simulink model "kalmannonlinear_noiseadded"  (R2019b)
settings: Solver=VariableStepAuto  StartTime=0.0  StopTime=10.0  RelTol=1e-3
libraries: sharedTrackingLibrary x9
settings Model: Creator=Bekircan Keceoglu  LastModifiedBy=Bekircan Keceoglu

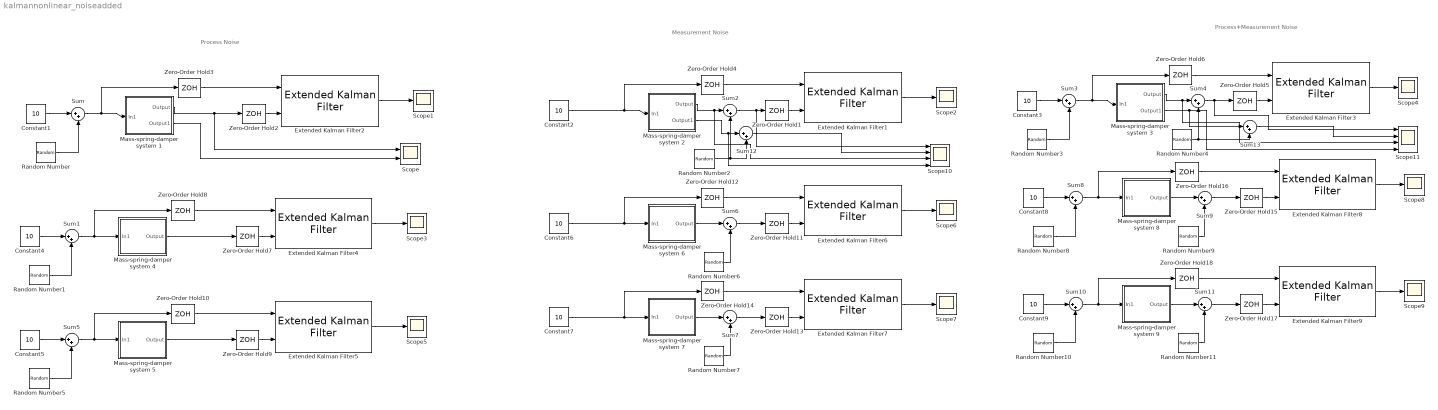
== system kalmannonlinear_noiseadded ==
  note: Process Noise
  note: Measurement Noise
  note: Process+Measurement Noise
  Constant{1..9} (9 alike) : Constant  Value=10
  Extended Kalman Filter1 : sharedTrackingLibrary/Extended Kalman Filter  StateTransitionFcn=myStateTransitionFcn  HasStateTransitionJacobianFcn=off  HasAdditiveProcessNoise=Additive  ProcessNoise=1  HasTimeVaryingProcessNoise=off  HasStateTransitionFcnExtraArgument=1  InitialState=[0 0]  InitialStateCovariance=1  MeasurementFcn1=myMeasurementFcn  HasMeasurementJacobianFcn1=off  HasMeasurementEnablePort1=off  HasAdditiveMeasurementNoise1=Additive  MeasurementNoise1=1  HasTimeVaryingMeasurementNoise1=off  HasMeasurementFcnExtraArgument1=0  MeasurementFcn2=myMeasurementFcn  HasMeasurementJacobianFcn2=off  HasMeasurementEnablePort2=off  HasAdditiveMeasurementNoise2=Additive  MeasurementNoise2=1  HasTimeVaryingMeasurementNoise2=off  HasMeasurementFcnExtraArgument2=0  MeasurementFcn3=myMeasurementFcn  HasMeasurementJacobianFcn3=off  HasMeasurementEnablePort3=off  HasAdditiveMeasurementNoise3=Additive  MeasurementNoise3=1  HasTimeVaryingMeasurementNoise3=off  HasMeasurementFcnExtraArgument3=0  MeasurementFcn4=myMeasurementFcn  HasMeasurementJacobianFcn4=off  HasMeasurementEnablePort4=off  HasAdditiveMeasurementNoise4=Additive  MeasurementNoise4=1  HasTimeVaryingMeasurementNoise4=off  HasMeasurementFcnExtraArgument4=0  MeasurementFcn5=myMeasurementFcn  HasMeasurementJacobianFcn5=off  HasMeasurementEnablePort5=off  HasAdditiveMeasurementNoise5=Additive  MeasurementNoise5=1  HasTimeVaryingMeasurementNoise5=off  HasMeasurementFcnExtraArgument5=0  EnableMultirate=off  StateTransitionFcnSampleTime=1  MeasurementFcn1SampleTime=1  MeasurementFcn2SampleTime=1  MeasurementFcn3SampleTime=1  MeasurementFcn4SampleTime=1  MeasurementFcn5SampleTime=1  UseCurrentEstimator=on  OutputStateCovariance=off  DataType=double  SampleTime=10e-3  NumberOfMeasurements=1
      settings: SourceProductName=Control System Toolbox  SourceProductBaseCode=CT
  Extended Kalman Filter2 : sharedTrackingLibrary/Extended Kalman Filter  StateTransitionFcn=myStateTransitionFcn  HasStateTransitionJacobianFcn=off  HasAdditiveProcessNoise=Additive  ProcessNoise=1  HasTimeVaryingProcessNoise=off  HasStateTransitionFcnExtraArgument=1  InitialState=[0 0]  InitialStateCovariance=1  MeasurementFcn1=myMeasurementFcn  HasMeasurementJacobianFcn1=off  HasMeasurementEnablePort1=off  HasAdditiveMeasurementNoise1=Additive  MeasurementNoise1=1  HasTimeVaryingMeasurementNoise1=off  HasMeasurementFcnExtraArgument1=0  MeasurementFcn2=myMeasurementFcn  HasMeasurementJacobianFcn2=off  HasMeasurementEnablePort2=off  HasAdditiveMeasurementNoise2=Additive  MeasurementNoise2=1  HasTimeVaryingMeasurementNoise2=off  HasMeasurementFcnExtraArgument2=0  MeasurementFcn3=myMeasurementFcn  HasMeasurementJacobianFcn3=off  HasMeasurementEnablePort3=off  HasAdditiveMeasurementNoise3=Additive  MeasurementNoise3=1  HasTimeVaryingMeasurementNoise3=off  HasMeasurementFcnExtraArgument3=0  MeasurementFcn4=myMeasurementFcn  HasMeasurementJacobianFcn4=off  HasMeasurementEnablePort4=off  HasAdditiveMeasurementNoise4=Additive  MeasurementNoise4=1  HasTimeVaryingMeasurementNoise4=off  HasMeasurementFcnExtraArgument4=0  MeasurementFcn5=myMeasurementFcn  HasMeasurementJacobianFcn5=off  HasMeasurementEnablePort5=off  HasAdditiveMeasurementNoise5=Additive  MeasurementNoise5=1  HasTimeVaryingMeasurementNoise5=off  HasMeasurementFcnExtraArgument5=0  EnableMultirate=off  StateTransitionFcnSampleTime=1  MeasurementFcn1SampleTime=1  MeasurementFcn2SampleTime=1  MeasurementFcn3SampleTime=1  MeasurementFcn4SampleTime=1  MeasurementFcn5SampleTime=1  UseCurrentEstimator=on  OutputStateCovariance=off  DataType=double  SampleTime=10e-3  NumberOfMeasurements=1
      settings: SourceProductName=Control System Toolbox  SourceProductBaseCode=CT
  Extended Kalman Filter3 : sharedTrackingLibrary/Extended Kalman Filter  StateTransitionFcn=myStateTransitionFcn  HasStateTransitionJacobianFcn=off  HasAdditiveProcessNoise=Additive  ProcessNoise=1  HasTimeVaryingProcessNoise=off  HasStateTransitionFcnExtraArgument=1  InitialState=[0 0]  InitialStateCovariance=1  MeasurementFcn1=myMeasurementFcn  HasMeasurementJacobianFcn1=off  HasMeasurementEnablePort1=off  HasAdditiveMeasurementNoise1=Additive  MeasurementNoise1=1  HasTimeVaryingMeasurementNoise1=off  HasMeasurementFcnExtraArgument1=0  MeasurementFcn2=myMeasurementFcn  HasMeasurementJacobianFcn2=off  HasMeasurementEnablePort2=off  HasAdditiveMeasurementNoise2=Additive  MeasurementNoise2=1  HasTimeVaryingMeasurementNoise2=off  HasMeasurementFcnExtraArgument2=0  MeasurementFcn3=myMeasurementFcn  HasMeasurementJacobianFcn3=off  HasMeasurementEnablePort3=off  HasAdditiveMeasurementNoise3=Additive  MeasurementNoise3=1  HasTimeVaryingMeasurementNoise3=off  HasMeasurementFcnExtraArgument3=0  MeasurementFcn4=myMeasurementFcn  HasMeasurementJacobianFcn4=off  HasMeasurementEnablePort4=off  HasAdditiveMeasurementNoise4=Additive  MeasurementNoise4=1  HasTimeVaryingMeasurementNoise4=off  HasMeasurementFcnExtraArgument4=0  MeasurementFcn5=myMeasurementFcn  HasMeasurementJacobianFcn5=off  HasMeasurementEnablePort5=off  HasAdditiveMeasurementNoise5=Additive  MeasurementNoise5=1  HasTimeVaryingMeasurementNoise5=off  HasMeasurementFcnExtraArgument5=0  EnableMultirate=off  StateTransitionFcnSampleTime=1  MeasurementFcn1SampleTime=1  MeasurementFcn2SampleTime=1  MeasurementFcn3SampleTime=1  MeasurementFcn4SampleTime=1  MeasurementFcn5SampleTime=1  UseCurrentEstimator=on  OutputStateCovariance=off  DataType=double  SampleTime=10e-3  NumberOfMeasurements=1
      settings: SourceProductName=Control System Toolbox  SourceProductBaseCode=CT
  Extended Kalman Filter4 : sharedTrackingLibrary/Extended Kalman Filter  StateTransitionFcn=myStateTransitionFcn  HasStateTransitionJacobianFcn=off  HasAdditiveProcessNoise=Additive  ProcessNoise=10  HasTimeVaryingProcessNoise=off  HasStateTransitionFcnExtraArgument=1  InitialState=[0 0]  InitialStateCovariance=1  MeasurementFcn1=myMeasurementFcn  HasMeasurementJacobianFcn1=off  HasMeasurementEnablePort1=off  HasAdditiveMeasurementNoise1=Additive  MeasurementNoise1=0.1  HasTimeVaryingMeasurementNoise1=off  HasMeasurementFcnExtraArgument1=0  MeasurementFcn2=myMeasurementFcn  HasMeasurementJacobianFcn2=off  HasMeasurementEnablePort2=off  HasAdditiveMeasurementNoise2=Additive  MeasurementNoise2=1  HasTimeVaryingMeasurementNoise2=off  HasMeasurementFcnExtraArgument2=0  MeasurementFcn3=myMeasurementFcn  HasMeasurementJacobianFcn3=off  HasMeasurementEnablePort3=off  HasAdditiveMeasurementNoise3=Additive  MeasurementNoise3=1  HasTimeVaryingMeasurementNoise3=off  HasMeasurementFcnExtraArgument3=0  MeasurementFcn4=myMeasurementFcn  HasMeasurementJacobianFcn4=off  HasMeasurementEnablePort4=off  HasAdditiveMeasurementNoise4=Additive  MeasurementNoise4=1  HasTimeVaryingMeasurementNoise4=off  HasMeasurementFcnExtraArgument4=0  MeasurementFcn5=myMeasurementFcn  HasMeasurementJacobianFcn5=off  HasMeasurementEnablePort5=off  HasAdditiveMeasurementNoise5=Additive  MeasurementNoise5=1  HasTimeVaryingMeasurementNoise5=off  HasMeasurementFcnExtraArgument5=0  EnableMultirate=off  StateTransitionFcnSampleTime=1  MeasurementFcn1SampleTime=1  MeasurementFcn2SampleTime=1  MeasurementFcn3SampleTime=1  MeasurementFcn4SampleTime=1  MeasurementFcn5SampleTime=1  UseCurrentEstimator=on  OutputStateCovariance=off  DataType=double  SampleTime=10e-3  NumberOfMeasurements=1
      settings: SourceProductName=Control System Toolbox  SourceProductBaseCode=CT
  Extended Kalman Filter5 : sharedTrackingLibrary/Extended Kalman Filter  StateTransitionFcn=myStateTransitionFcn  HasStateTransitionJacobianFcn=off  HasAdditiveProcessNoise=Additive  ProcessNoise=0.1  HasTimeVaryingProcessNoise=off  HasStateTransitionFcnExtraArgument=1  InitialState=[0 0]  InitialStateCovariance=1  MeasurementFcn1=myMeasurementFcn  HasMeasurementJacobianFcn1=off  HasMeasurementEnablePort1=off  HasAdditiveMeasurementNoise1=Additive  MeasurementNoise1=10  HasTimeVaryingMeasurementNoise1=off  HasMeasurementFcnExtraArgument1=0  MeasurementFcn2=myMeasurementFcn  HasMeasurementJacobianFcn2=off  HasMeasurementEnablePort2=off  HasAdditiveMeasurementNoise2=Additive  MeasurementNoise2=1  HasTimeVaryingMeasurementNoise2=off  HasMeasurementFcnExtraArgument2=0  MeasurementFcn3=myMeasurementFcn  HasMeasurementJacobianFcn3=off  HasMeasurementEnablePort3=off  HasAdditiveMeasurementNoise3=Additive  MeasurementNoise3=1  HasTimeVaryingMeasurementNoise3=off  HasMeasurementFcnExtraArgument3=0  MeasurementFcn4=myMeasurementFcn  HasMeasurementJacobianFcn4=off  HasMeasurementEnablePort4=off  HasAdditiveMeasurementNoise4=Additive  MeasurementNoise4=1  HasTimeVaryingMeasurementNoise4=off  HasMeasurementFcnExtraArgument4=0  MeasurementFcn5=myMeasurementFcn  HasMeasurementJacobianFcn5=off  HasMeasurementEnablePort5=off  HasAdditiveMeasurementNoise5=Additive  MeasurementNoise5=1  HasTimeVaryingMeasurementNoise5=off  HasMeasurementFcnExtraArgument5=0  EnableMultirate=off  StateTransitionFcnSampleTime=1  MeasurementFcn1SampleTime=1  MeasurementFcn2SampleTime=1  MeasurementFcn3SampleTime=1  MeasurementFcn4SampleTime=1  MeasurementFcn5SampleTime=1  UseCurrentEstimator=on  OutputStateCovariance=off  DataType=double  SampleTime=10e-3  NumberOfMeasurements=1
      settings: SourceProductName=Control System Toolbox  SourceProductBaseCode=CT
  Extended Kalman Filter6 : sharedTrackingLibrary/Extended Kalman Filter  StateTransitionFcn=myStateTransitionFcn  HasStateTransitionJacobianFcn=off  HasAdditiveProcessNoise=Additive  ProcessNoise=10  HasTimeVaryingProcessNoise=off  HasStateTransitionFcnExtraArgument=1  InitialState=[0 0]  InitialStateCovariance=1  MeasurementFcn1=myMeasurementFcn  HasMeasurementJacobianFcn1=off  HasMeasurementEnablePort1=off  HasAdditiveMeasurementNoise1=Additive  MeasurementNoise1=0.1  HasTimeVaryingMeasurementNoise1=off  HasMeasurementFcnExtraArgument1=0  MeasurementFcn2=myMeasurementFcn  HasMeasurementJacobianFcn2=off  HasMeasurementEnablePort2=off  HasAdditiveMeasurementNoise2=Additive  MeasurementNoise2=1  HasTimeVaryingMeasurementNoise2=off  HasMeasurementFcnExtraArgument2=0  MeasurementFcn3=myMeasurementFcn  HasMeasurementJacobianFcn3=off  HasMeasurementEnablePort3=off  HasAdditiveMeasurementNoise3=Additive  MeasurementNoise3=1  HasTimeVaryingMeasurementNoise3=off  HasMeasurementFcnExtraArgument3=0  MeasurementFcn4=myMeasurementFcn  HasMeasurementJacobianFcn4=off  HasMeasurementEnablePort4=off  HasAdditiveMeasurementNoise4=Additive  MeasurementNoise4=1  HasTimeVaryingMeasurementNoise4=off  HasMeasurementFcnExtraArgument4=0  MeasurementFcn5=myMeasurementFcn  HasMeasurementJacobianFcn5=off  HasMeasurementEnablePort5=off  HasAdditiveMeasurementNoise5=Additive  MeasurementNoise5=1  HasTimeVaryingMeasurementNoise5=off  HasMeasurementFcnExtraArgument5=0  EnableMultirate=off  StateTransitionFcnSampleTime=1  MeasurementFcn1SampleTime=1  MeasurementFcn2SampleTime=1  MeasurementFcn3SampleTime=1  MeasurementFcn4SampleTime=1  MeasurementFcn5SampleTime=1  UseCurrentEstimator=on  OutputStateCovariance=off  DataType=double  SampleTime=10e-3  NumberOfMeasurements=1
      settings: SourceProductName=Control System Toolbox  SourceProductBaseCode=CT
  Extended Kalman Filter7 : sharedTrackingLibrary/Extended Kalman Filter  StateTransitionFcn=myStateTransitionFcn  HasStateTransitionJacobianFcn=off  HasAdditiveProcessNoise=Additive  ProcessNoise=0.1  HasTimeVaryingProcessNoise=off  HasStateTransitionFcnExtraArgument=1  InitialState=[0 0]  InitialStateCovariance=1  MeasurementFcn1=myMeasurementFcn  HasMeasurementJacobianFcn1=off  HasMeasurementEnablePort1=off  HasAdditiveMeasurementNoise1=Additive  MeasurementNoise1=10  HasTimeVaryingMeasurementNoise1=off  HasMeasurementFcnExtraArgument1=0  MeasurementFcn2=myMeasurementFcn  HasMeasurementJacobianFcn2=off  HasMeasurementEnablePort2=off  HasAdditiveMeasurementNoise2=Additive  MeasurementNoise2=1  HasTimeVaryingMeasurementNoise2=off  HasMeasurementFcnExtraArgument2=0  MeasurementFcn3=myMeasurementFcn  HasMeasurementJacobianFcn3=off  HasMeasurementEnablePort3=off  HasAdditiveMeasurementNoise3=Additive  MeasurementNoise3=1  HasTimeVaryingMeasurementNoise3=off  HasMeasurementFcnExtraArgument3=0  MeasurementFcn4=myMeasurementFcn  HasMeasurementJacobianFcn4=off  HasMeasurementEnablePort4=off  HasAdditiveMeasurementNoise4=Additive  MeasurementNoise4=1  HasTimeVaryingMeasurementNoise4=off  HasMeasurementFcnExtraArgument4=0  MeasurementFcn5=myMeasurementFcn  HasMeasurementJacobianFcn5=off  HasMeasurementEnablePort5=off  HasAdditiveMeasurementNoise5=Additive  MeasurementNoise5=1  HasTimeVaryingMeasurementNoise5=off  HasMeasurementFcnExtraArgument5=0  EnableMultirate=off  StateTransitionFcnSampleTime=1  MeasurementFcn1SampleTime=1  MeasurementFcn2SampleTime=1  MeasurementFcn3SampleTime=1  MeasurementFcn4SampleTime=1  MeasurementFcn5SampleTime=1  UseCurrentEstimator=on  OutputStateCovariance=off  DataType=double  SampleTime=10e-3  NumberOfMeasurements=1
      settings: SourceProductName=Control System Toolbox  SourceProductBaseCode=CT
  Extended Kalman Filter8 : sharedTrackingLibrary/Extended Kalman Filter  StateTransitionFcn=myStateTransitionFcn  HasStateTransitionJacobianFcn=off  HasAdditiveProcessNoise=Additive  ProcessNoise=10  HasTimeVaryingProcessNoise=off  HasStateTransitionFcnExtraArgument=1  InitialState=[0 0]  InitialStateCovariance=1  MeasurementFcn1=myMeasurementFcn  HasMeasurementJacobianFcn1=off  HasMeasurementEnablePort1=off  HasAdditiveMeasurementNoise1=Additive  MeasurementNoise1=0.1  HasTimeVaryingMeasurementNoise1=off  HasMeasurementFcnExtraArgument1=0  MeasurementFcn2=myMeasurementFcn  HasMeasurementJacobianFcn2=off  HasMeasurementEnablePort2=off  HasAdditiveMeasurementNoise2=Additive  MeasurementNoise2=1  HasTimeVaryingMeasurementNoise2=off  HasMeasurementFcnExtraArgument2=0  MeasurementFcn3=myMeasurementFcn  HasMeasurementJacobianFcn3=off  HasMeasurementEnablePort3=off  HasAdditiveMeasurementNoise3=Additive  MeasurementNoise3=1  HasTimeVaryingMeasurementNoise3=off  HasMeasurementFcnExtraArgument3=0  MeasurementFcn4=myMeasurementFcn  HasMeasurementJacobianFcn4=off  HasMeasurementEnablePort4=off  HasAdditiveMeasurementNoise4=Additive  MeasurementNoise4=1  HasTimeVaryingMeasurementNoise4=off  HasMeasurementFcnExtraArgument4=0  MeasurementFcn5=myMeasurementFcn  HasMeasurementJacobianFcn5=off  HasMeasurementEnablePort5=off  HasAdditiveMeasurementNoise5=Additive  MeasurementNoise5=1  HasTimeVaryingMeasurementNoise5=off  HasMeasurementFcnExtraArgument5=0  EnableMultirate=off  StateTransitionFcnSampleTime=1  MeasurementFcn1SampleTime=1  MeasurementFcn2SampleTime=1  MeasurementFcn3SampleTime=1  MeasurementFcn4SampleTime=1  MeasurementFcn5SampleTime=1  UseCurrentEstimator=on  OutputStateCovariance=off  DataType=double  SampleTime=10e-3  NumberOfMeasurements=1
      settings: SourceProductName=Control System Toolbox  SourceProductBaseCode=CT
  Extended Kalman Filter9 : sharedTrackingLibrary/Extended Kalman Filter  StateTransitionFcn=myStateTransitionFcn  HasStateTransitionJacobianFcn=off  HasAdditiveProcessNoise=Additive  ProcessNoise=0.1  HasTimeVaryingProcessNoise=off  HasStateTransitionFcnExtraArgument=1  InitialState=[0 0]  InitialStateCovariance=1  MeasurementFcn1=myMeasurementFcn  HasMeasurementJacobianFcn1=off  HasMeasurementEnablePort1=off  HasAdditiveMeasurementNoise1=Additive  MeasurementNoise1=10  HasTimeVaryingMeasurementNoise1=off  HasMeasurementFcnExtraArgument1=0  MeasurementFcn2=myMeasurementFcn  HasMeasurementJacobianFcn2=off  HasMeasurementEnablePort2=off  HasAdditiveMeasurementNoise2=Additive  MeasurementNoise2=1  HasTimeVaryingMeasurementNoise2=off  HasMeasurementFcnExtraArgument2=0  MeasurementFcn3=myMeasurementFcn  HasMeasurementJacobianFcn3=off  HasMeasurementEnablePort3=off  HasAdditiveMeasurementNoise3=Additive  MeasurementNoise3=1  HasTimeVaryingMeasurementNoise3=off  HasMeasurementFcnExtraArgument3=0  MeasurementFcn4=myMeasurementFcn  HasMeasurementJacobianFcn4=off  HasMeasurementEnablePort4=off  HasAdditiveMeasurementNoise4=Additive  MeasurementNoise4=1  HasTimeVaryingMeasurementNoise4=off  HasMeasurementFcnExtraArgument4=0  MeasurementFcn5=myMeasurementFcn  HasMeasurementJacobianFcn5=off  HasMeasurementEnablePort5=off  HasAdditiveMeasurementNoise5=Additive  MeasurementNoise5=1  HasTimeVaryingMeasurementNoise5=off  HasMeasurementFcnExtraArgument5=0  EnableMultirate=off  StateTransitionFcnSampleTime=1  MeasurementFcn1SampleTime=1  MeasurementFcn2SampleTime=1  MeasurementFcn3SampleTime=1  MeasurementFcn4SampleTime=1  MeasurementFcn5SampleTime=1  UseCurrentEstimator=on  OutputStateCovariance=off  DataType=double  SampleTime=10e-3  NumberOfMeasurements=1
      settings: SourceProductName=Control System Toolbox  SourceProductBaseCode=CT
  Mass-spring-damper system 1 : Subsystem
  Mass-spring-damper system 2 : Subsystem
  Mass-spring-damper system 3 : Subsystem
  Mass-spring-damper system 4 : Subsystem
  Mass-spring-damper system 5 : Subsystem
  Mass-spring-damper system 6 : Subsystem
  Mass-spring-damper system 7 : Subsystem
  Mass-spring-damper system 8 : Subsystem
  Mass-spring-damper system 9 : Subsystem
  Random Number{,1..11} (12 alike) : RandomNumber  Mean=0.1  Variance=0.1  SampleTime=0.1
  Scope : Scope  NumInputPorts=2
  Scope{1..9} (9 alike) : Scope
  Scope10 : Scope  NumInputPorts=4
  Scope11 : Scope  NumInputPorts=4
  Sum{,1..13} (14 alike) : Sum  Inputs=|++
  Zero-Order Hold{1..18} (18 alike) : ZeroOrderHold  SampleTime=10e-3
  wires:
  Extended Kalman Filter2/1 -> Scope1/1
  Mass-spring-damper system 1/1(Output) -> Scope/1, Zero-Order Hold2/1
  Constant1/1 -> Sum/1
  Sum/1 -> Zero-Order Hold3/1, Mass-spring-damper system 1/1(In1)
  Zero-Order Hold3/1 -> Extended Kalman Filter2/1
  Zero-Order Hold2/1 -> Extended Kalman Filter2/2
  Random Number/1 -> Sum/2
  Zero-Order Hold4/1 -> Extended Kalman Filter1/1
  Zero-Order Hold1/1 -> Extended Kalman Filter1/2
  Extended Kalman Filter1/1 -> Scope2/1
  Constant2/1 -> Zero-Order Hold4/1, Mass-spring-damper system 2/1(In1)
  Mass-spring-damper system 2/1(Output) -> Scope10/3, Sum2/1
  Sum2/1 -> Scope10/1, Zero-Order Hold1/1
  Random Number2/1 -> Sum12/2, Sum2/2
  Random Number3/1 -> Sum3/2
  Constant3/1 -> Sum3/1
  Zero-Order Hold5/1 -> Extended Kalman Filter3/2
  Zero-Order Hold6/1 -> Extended Kalman Filter3/1
  Mass-spring-damper system 3/1(Output) -> Scope11/3, Sum4/1
  Random Number4/1 -> Sum13/2, Sum4/2
  Sum3/1 -> Zero-Order Hold6/1, Mass-spring-damper system 3/1(In1)
  Sum4/1 -> Scope11/1, Zero-Order Hold5/1
  Extended Kalman Filter3/1 -> Scope4/1
  Zero-Order Hold8/1 -> Extended Kalman Filter4/1
  Zero-Order Hold7/1 -> Extended Kalman Filter4/2
  Mass-spring-damper system 4/1(Output) -> Zero-Order Hold7/1
  Random Number1/1 -> Sum1/2
  Constant4/1 -> Sum1/1
  Extended Kalman Filter4/1 -> Scope3/1
  Sum1/1 -> Zero-Order Hold8/1, Mass-spring-damper system 4/1(In1)
  Zero-Order Hold10/1 -> Extended Kalman Filter5/1
  Zero-Order Hold9/1 -> Extended Kalman Filter5/2
  Mass-spring-damper system 5/1(Output) -> Zero-Order Hold9/1
  Random Number5/1 -> Sum5/2
  Constant5/1 -> Sum5/1
  Extended Kalman Filter5/1 -> Scope5/1
  Sum5/1 -> Zero-Order Hold10/1, Mass-spring-damper system 5/1(In1)
  Zero-Order Hold11/1 -> Extended Kalman Filter6/2
  Zero-Order Hold12/1 -> Extended Kalman Filter6/1
  Mass-spring-damper system 6/1(Output) -> Sum6/1
  Random Number6/1 -> Sum6/2
  Extended Kalman Filter6/1 -> Scope6/1
  Sum6/1 -> Zero-Order Hold11/1
  Constant6/1 -> Zero-Order Hold12/1, Mass-spring-damper system 6/1(In1)
  Zero-Order Hold13/1 -> Extended Kalman Filter7/2
  Zero-Order Hold14/1 -> Extended Kalman Filter7/1
  Mass-spring-damper system 7/1(Output) -> Sum7/1
  Random Number7/1 -> Sum7/2
  Extended Kalman Filter7/1 -> Scope7/1
  Sum7/1 -> Zero-Order Hold13/1
  Constant7/1 -> Zero-Order Hold14/1, Mass-spring-damper system 7/1(In1)
  Sum9/1 -> Zero-Order Hold15/1
  Random Number9/1 -> Sum9/2
  Constant8/1 -> Sum8/1
  Mass-spring-damper system 8/1(Output) -> Sum9/1
  Zero-Order Hold16/1 -> Extended Kalman Filter8/1
  Sum8/1 -> Zero-Order Hold16/1, Mass-spring-damper system 8/1(In1)
  Zero-Order Hold15/1 -> Extended Kalman Filter8/2
  Random Number8/1 -> Sum8/2
  Extended Kalman Filter8/1 -> Scope8/1
  Sum11/1 -> Zero-Order Hold17/1
  Random Number11/1 -> Sum11/2
  Constant9/1 -> Sum10/1
  Mass-spring-damper system 9/1(Output) -> Sum11/1
  Zero-Order Hold18/1 -> Extended Kalman Filter9/1
  Sum10/1 -> Zero-Order Hold18/1, Mass-spring-damper system 9/1(In1)
  Zero-Order Hold17/1 -> Extended Kalman Filter9/2
  Random Number10/1 -> Sum10/2
  Extended Kalman Filter9/1 -> Scope9/1
  Mass-spring-damper system 1/2(Output1) -> Scope/2
  Mass-spring-damper system 2/2(Output1) -> Scope10/4, Sum12/1
  Sum12/1 -> Scope10/2
  Mass-spring-damper system 3/2(Output1) -> Scope11/4, Sum13/1
  Sum13/1 -> Scope11/2

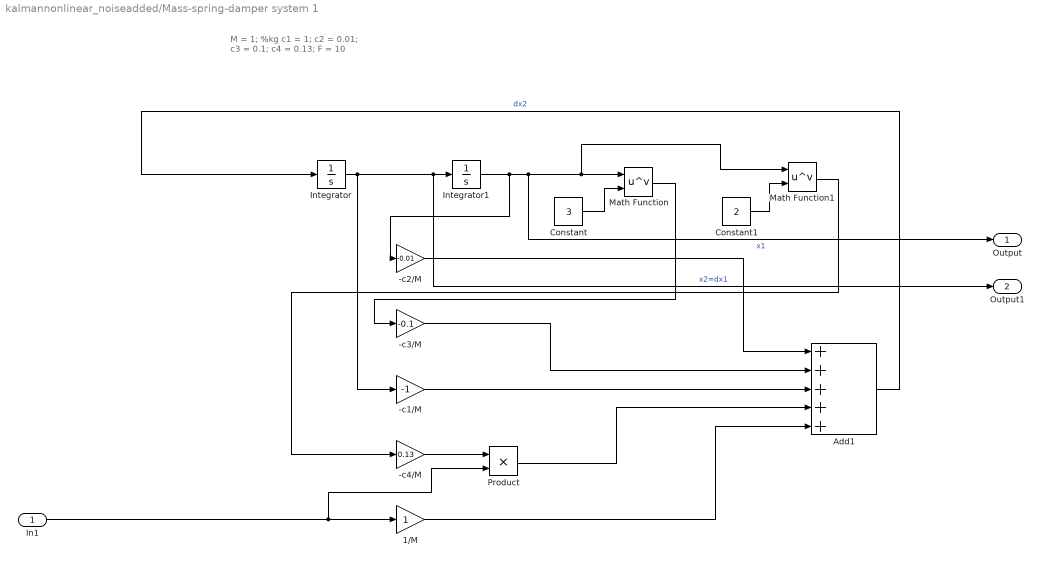
== system kalmannonlinear_noiseadded/Mass-spring-damper system 1 ==
  note: M  = 1; %kg
      | c1 = 1;
      | c2 = 0.01;
      | c3 = 0.1;
      | c4 = 0.13;
      | F  = 10
  In1 : Inport
  -c1/M : Gain  Gain=-1
  -c2/M : Gain  Gain=-0.01
  -c3/M : Gain  Gain=-0.1
  -c4/M : Gain  Gain=0.13
  1/M : Gain
  Add1 : Sum  Inputs=+++++
  Constant : Constant  Value=3
  Constant1 : Constant  Value=2
  Integrator : Integrator  InitialCondition=5
  Integrator1 : Integrator
  Math Function : Math  Operator=pow  SignedPower=off  SaturateOnIntegerOverflow=on
  Math Function1 : Math  Operator=pow  SignedPower=off  SaturateOnIntegerOverflow=on
  Product : Product
  Output : Outport
  Output1 : Outport  Port=2
  wires:
  Integrator1/1 -> -c2/M/1, Output/1, Math Function1/1, Math Function/1  "x1"
  Math Function/1 -> -c3/M/1
  Constant/1 -> Math Function/2
  -c3/M/1 -> Add1/2
  Product/1 -> Add1/4
  -c1/M/1 -> Add1/3
  -c4/M/1 -> Product/1
  Math Function1/1 -> -c4/M/1
  Constant1/1 -> Math Function1/2
  -c2/M/1 -> Add1/1
  In1/1 -> Product/2, 1/M/1
  Integrator/1 -> -c1/M/1, Output1/1, Integrator1/1  "x2=dx1"
  Add1/1 -> Integrator/1  "dx2"
  1/M/1 -> Add1/5

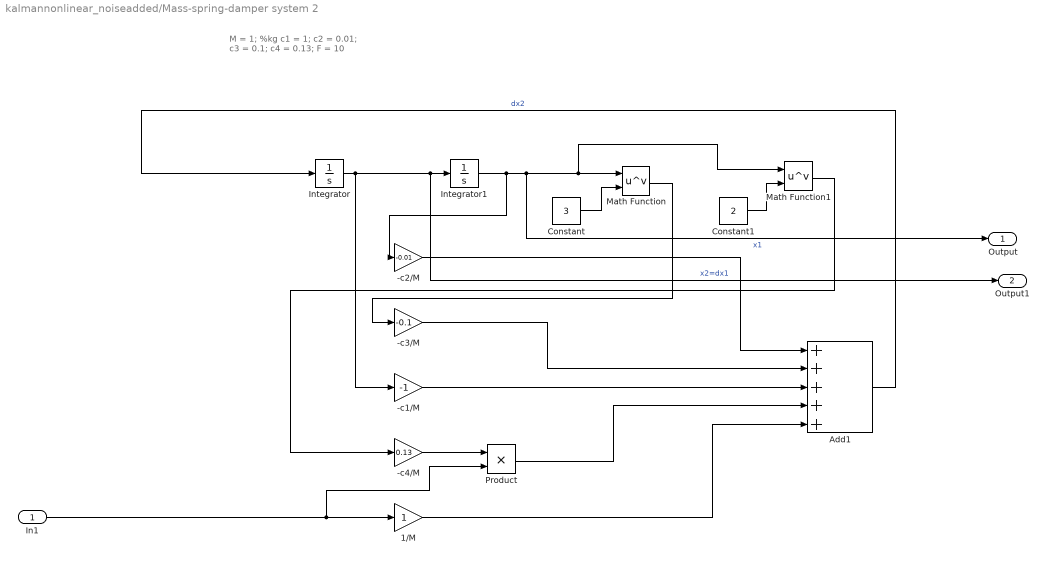
== system kalmannonlinear_noiseadded/Mass-spring-damper system 2 ==
  note: M  = 1; %kg
      | c1 = 1;
      | c2 = 0.01;
      | c3 = 0.1;
      | c4 = 0.13;
      | F  = 10
  In1 : Inport
  -c1/M : Gain  Gain=-1
  -c2/M : Gain  Gain=-0.01
  -c3/M : Gain  Gain=-0.1
  -c4/M : Gain  Gain=0.13
  1/M : Gain
  Add1 : Sum  Inputs=+++++
  Constant : Constant  Value=3
  Constant1 : Constant  Value=2
  Integrator : Integrator  InitialCondition=5
  Integrator1 : Integrator
  Math Function : Math  Operator=pow  SignedPower=off  SaturateOnIntegerOverflow=on
  Math Function1 : Math  Operator=pow  SignedPower=off  SaturateOnIntegerOverflow=on
  Product : Product
  Output : Outport
  Output1 : Outport  Port=2
  wires:
  Integrator1/1 -> -c2/M/1, Output/1, Math Function1/1, Math Function/1  "x1"
  Math Function/1 -> -c3/M/1
  Constant/1 -> Math Function/2
  -c3/M/1 -> Add1/2
  Product/1 -> Add1/4
  -c1/M/1 -> Add1/3
  -c4/M/1 -> Product/1
  Math Function1/1 -> -c4/M/1
  Constant1/1 -> Math Function1/2
  -c2/M/1 -> Add1/1
  In1/1 -> Product/2, 1/M/1
  Integrator/1 -> -c1/M/1, Output1/1, Integrator1/1  "x2=dx1"
  Add1/1 -> Integrator/1  "dx2"
  1/M/1 -> Add1/5

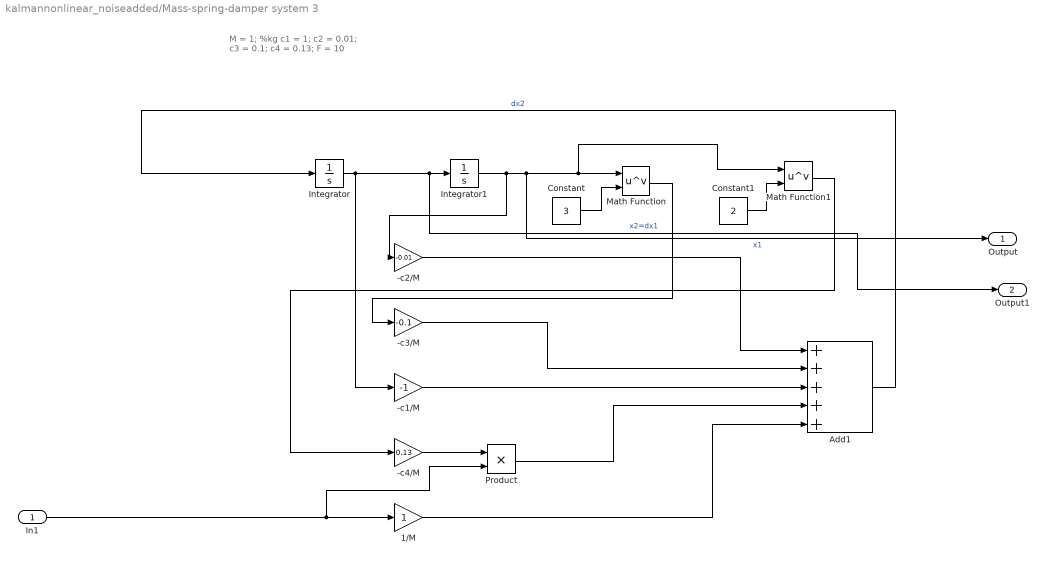
== system kalmannonlinear_noiseadded/Mass-spring-damper system 3 ==
  note: M  = 1; %kg
      | c1 = 1;
      | c2 = 0.01;
      | c3 = 0.1;
      | c4 = 0.13;
      | F  = 10
  In1 : Inport
  -c1/M : Gain  Gain=-1
  -c2/M : Gain  Gain=-0.01
  -c3/M : Gain  Gain=-0.1
  -c4/M : Gain  Gain=0.13
  1/M : Gain
  Add1 : Sum  Inputs=+++++
  Constant : Constant  Value=3
  Constant1 : Constant  Value=2
  Integrator : Integrator  InitialCondition=5
  Integrator1 : Integrator
  Math Function : Math  Operator=pow  SignedPower=off  SaturateOnIntegerOverflow=on
  Math Function1 : Math  Operator=pow  SignedPower=off  SaturateOnIntegerOverflow=on
  Product : Product
  Output : Outport
  Output1 : Outport  Port=2
  wires:
  Integrator1/1 -> -c2/M/1, Output/1, Math Function1/1, Math Function/1  "x1"
  Math Function/1 -> -c3/M/1
  Constant/1 -> Math Function/2
  -c3/M/1 -> Add1/2
  Product/1 -> Add1/4
  -c1/M/1 -> Add1/3
  -c4/M/1 -> Product/1
  Math Function1/1 -> -c4/M/1
  Constant1/1 -> Math Function1/2
  -c2/M/1 -> Add1/1
  In1/1 -> Product/2, 1/M/1
  Integrator/1 -> -c1/M/1, Output1/1, Integrator1/1  "x2=dx1"
  Add1/1 -> Integrator/1  "dx2"
  1/M/1 -> Add1/5

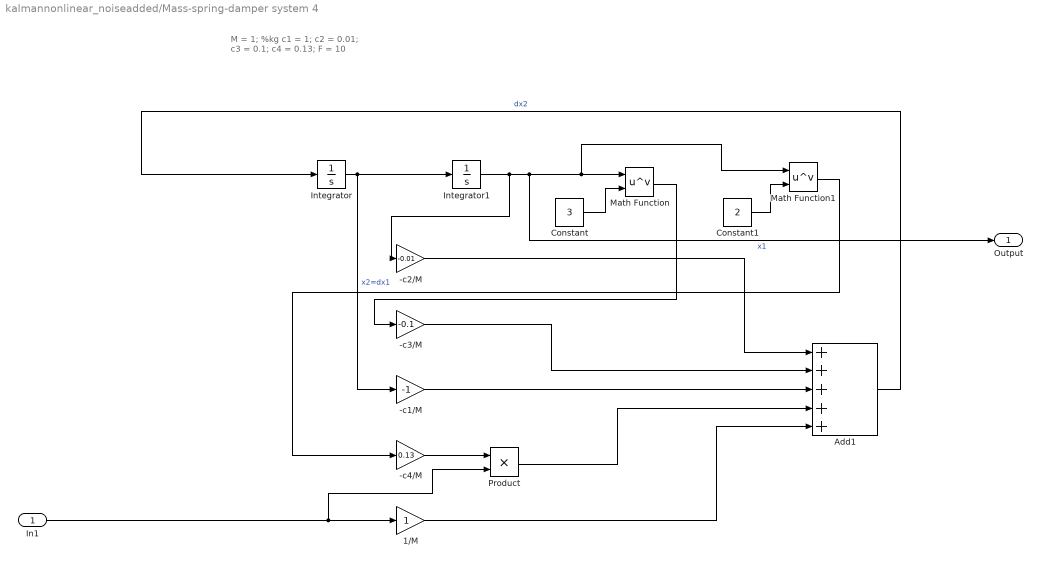
== system kalmannonlinear_noiseadded/Mass-spring-damper system 4 ==
  note: M  = 1; %kg
      | c1 = 1;
      | c2 = 0.01;
      | c3 = 0.1;
      | c4 = 0.13;
      | F  = 10
  In1 : Inport
  -c1/M : Gain  Gain=-1
  -c2/M : Gain  Gain=-0.01
  -c3/M : Gain  Gain=-0.1
  -c4/M : Gain  Gain=0.13
  1/M : Gain
  Add1 : Sum  Inputs=+++++
  Constant : Constant  Value=3
  Constant1 : Constant  Value=2
  Integrator : Integrator  InitialCondition=5
  Integrator1 : Integrator
  Math Function : Math  Operator=pow  SignedPower=off  SaturateOnIntegerOverflow=on
  Math Function1 : Math  Operator=pow  SignedPower=off  SaturateOnIntegerOverflow=on
  Product : Product
  Output : Outport
  wires:
  Integrator1/1 -> -c2/M/1, Output/1, Math Function1/1, Math Function/1  "x1"
  Math Function/1 -> -c3/M/1
  Constant/1 -> Math Function/2
  -c3/M/1 -> Add1/2
  Product/1 -> Add1/4
  -c1/M/1 -> Add1/3
  -c4/M/1 -> Product/1
  Math Function1/1 -> -c4/M/1
  Constant1/1 -> Math Function1/2
  -c2/M/1 -> Add1/1
  In1/1 -> Product/2, 1/M/1
  Integrator/1 -> -c1/M/1, Integrator1/1  "x2=dx1"
  Add1/1 -> Integrator/1  "dx2"
  1/M/1 -> Add1/5

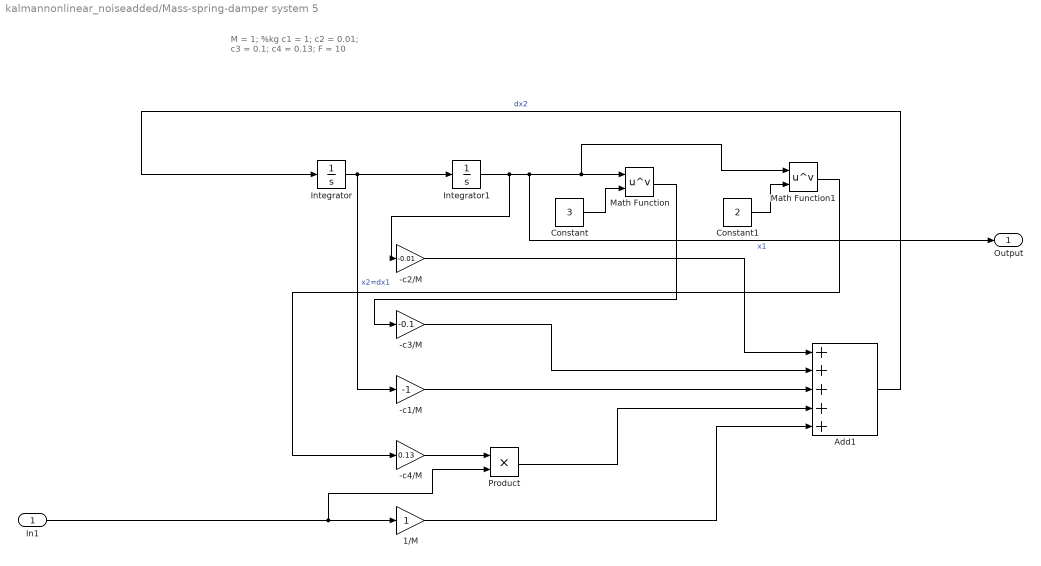
== system kalmannonlinear_noiseadded/Mass-spring-damper system 5 ==
  note: M  = 1; %kg
      | c1 = 1;
      | c2 = 0.01;
      | c3 = 0.1;
      | c4 = 0.13;
      | F  = 10
  In1 : Inport
  -c1/M : Gain  Gain=-1
  -c2/M : Gain  Gain=-0.01
  -c3/M : Gain  Gain=-0.1
  -c4/M : Gain  Gain=0.13
  1/M : Gain
  Add1 : Sum  Inputs=+++++
  Constant : Constant  Value=3
  Constant1 : Constant  Value=2
  Integrator : Integrator  InitialCondition=5
  Integrator1 : Integrator
  Math Function : Math  Operator=pow  SignedPower=off  SaturateOnIntegerOverflow=on
  Math Function1 : Math  Operator=pow  SignedPower=off  SaturateOnIntegerOverflow=on
  Product : Product
  Output : Outport
  wires:
  Integrator1/1 -> -c2/M/1, Output/1, Math Function1/1, Math Function/1  "x1"
  Math Function/1 -> -c3/M/1
  Constant/1 -> Math Function/2
  -c3/M/1 -> Add1/2
  Product/1 -> Add1/4
  -c1/M/1 -> Add1/3
  -c4/M/1 -> Product/1
  Math Function1/1 -> -c4/M/1
  Constant1/1 -> Math Function1/2
  -c2/M/1 -> Add1/1
  In1/1 -> Product/2, 1/M/1
  Integrator/1 -> -c1/M/1, Integrator1/1  "x2=dx1"
  Add1/1 -> Integrator/1  "dx2"
  1/M/1 -> Add1/5

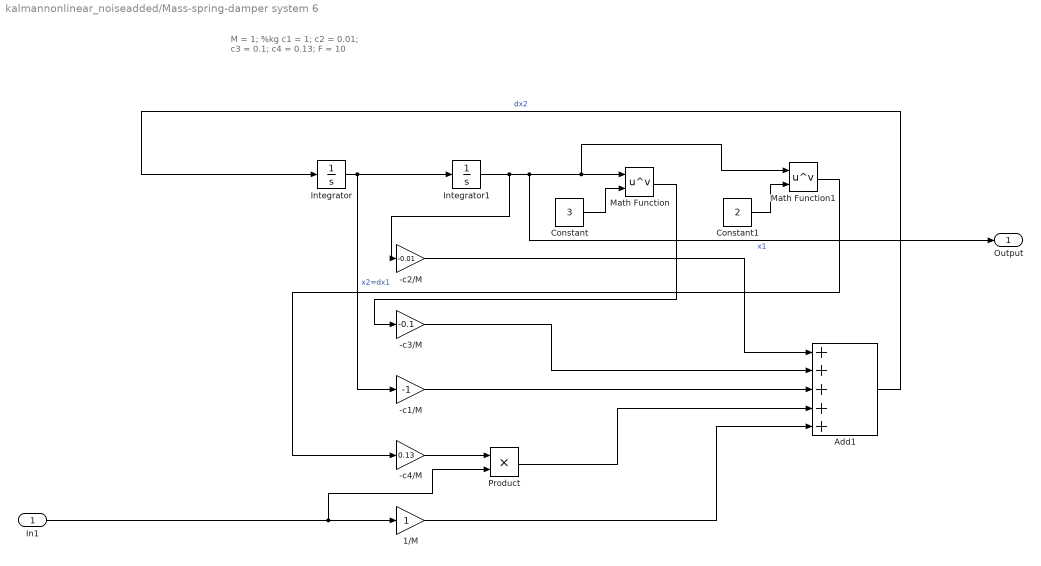
== system kalmannonlinear_noiseadded/Mass-spring-damper system 6 ==
  note: M  = 1; %kg
      | c1 = 1;
      | c2 = 0.01;
      | c3 = 0.1;
      | c4 = 0.13;
      | F  = 10
  In1 : Inport
  -c1/M : Gain  Gain=-1
  -c2/M : Gain  Gain=-0.01
  -c3/M : Gain  Gain=-0.1
  -c4/M : Gain  Gain=0.13
  1/M : Gain
  Add1 : Sum  Inputs=+++++
  Constant : Constant  Value=3
  Constant1 : Constant  Value=2
  Integrator : Integrator  InitialCondition=5
  Integrator1 : Integrator
  Math Function : Math  Operator=pow  SignedPower=off  SaturateOnIntegerOverflow=on
  Math Function1 : Math  Operator=pow  SignedPower=off  SaturateOnIntegerOverflow=on
  Product : Product
  Output : Outport
  wires:
  Integrator1/1 -> -c2/M/1, Output/1, Math Function1/1, Math Function/1  "x1"
  Math Function/1 -> -c3/M/1
  Constant/1 -> Math Function/2
  -c3/M/1 -> Add1/2
  Product/1 -> Add1/4
  -c1/M/1 -> Add1/3
  -c4/M/1 -> Product/1
  Math Function1/1 -> -c4/M/1
  Constant1/1 -> Math Function1/2
  -c2/M/1 -> Add1/1
  In1/1 -> Product/2, 1/M/1
  Integrator/1 -> -c1/M/1, Integrator1/1  "x2=dx1"
  Add1/1 -> Integrator/1  "dx2"
  1/M/1 -> Add1/5

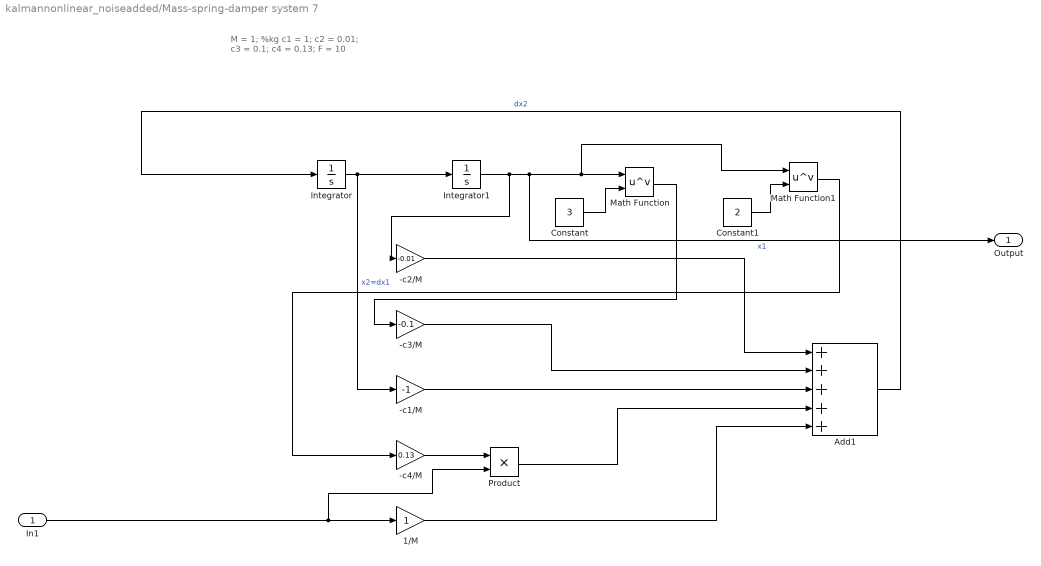
== system kalmannonlinear_noiseadded/Mass-spring-damper system 7 ==
  note: M  = 1; %kg
      | c1 = 1;
      | c2 = 0.01;
      | c3 = 0.1;
      | c4 = 0.13;
      | F  = 10
  In1 : Inport
  -c1/M : Gain  Gain=-1
  -c2/M : Gain  Gain=-0.01
  -c3/M : Gain  Gain=-0.1
  -c4/M : Gain  Gain=0.13
  1/M : Gain
  Add1 : Sum  Inputs=+++++
  Constant : Constant  Value=3
  Constant1 : Constant  Value=2
  Integrator : Integrator  InitialCondition=5
  Integrator1 : Integrator
  Math Function : Math  Operator=pow  SignedPower=off  SaturateOnIntegerOverflow=on
  Math Function1 : Math  Operator=pow  SignedPower=off  SaturateOnIntegerOverflow=on
  Product : Product
  Output : Outport
  wires:
  Integrator1/1 -> -c2/M/1, Output/1, Math Function1/1, Math Function/1  "x1"
  Math Function/1 -> -c3/M/1
  Constant/1 -> Math Function/2
  -c3/M/1 -> Add1/2
  Product/1 -> Add1/4
  -c1/M/1 -> Add1/3
  -c4/M/1 -> Product/1
  Math Function1/1 -> -c4/M/1
  Constant1/1 -> Math Function1/2
  -c2/M/1 -> Add1/1
  In1/1 -> Product/2, 1/M/1
  Integrator/1 -> -c1/M/1, Integrator1/1  "x2=dx1"
  Add1/1 -> Integrator/1  "dx2"
  1/M/1 -> Add1/5

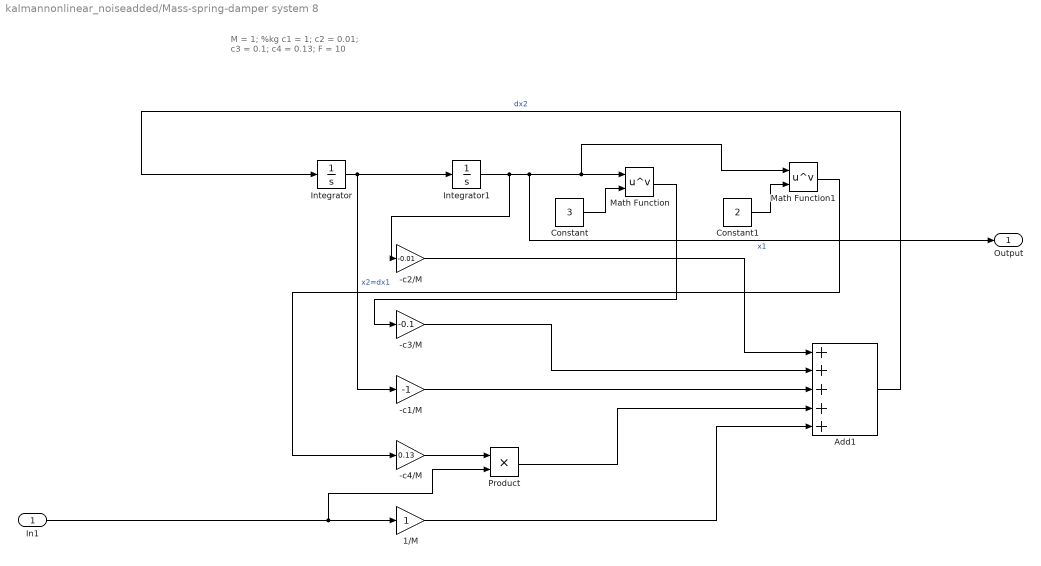
== system kalmannonlinear_noiseadded/Mass-spring-damper system 8 ==
  note: M  = 1; %kg
      | c1 = 1;
      | c2 = 0.01;
      | c3 = 0.1;
      | c4 = 0.13;
      | F  = 10
  In1 : Inport
  -c1/M : Gain  Gain=-1
  -c2/M : Gain  Gain=-0.01
  -c3/M : Gain  Gain=-0.1
  -c4/M : Gain  Gain=0.13
  1/M : Gain
  Add1 : Sum  Inputs=+++++
  Constant : Constant  Value=3
  Constant1 : Constant  Value=2
  Integrator : Integrator  InitialCondition=5
  Integrator1 : Integrator
  Math Function : Math  Operator=pow  SignedPower=off  SaturateOnIntegerOverflow=on
  Math Function1 : Math  Operator=pow  SignedPower=off  SaturateOnIntegerOverflow=on
  Product : Product
  Output : Outport
  wires:
  Integrator1/1 -> -c2/M/1, Output/1, Math Function1/1, Math Function/1  "x1"
  Math Function/1 -> -c3/M/1
  Constant/1 -> Math Function/2
  -c3/M/1 -> Add1/2
  Product/1 -> Add1/4
  -c1/M/1 -> Add1/3
  -c4/M/1 -> Product/1
  Math Function1/1 -> -c4/M/1
  Constant1/1 -> Math Function1/2
  -c2/M/1 -> Add1/1
  In1/1 -> Product/2, 1/M/1
  Integrator/1 -> -c1/M/1, Integrator1/1  "x2=dx1"
  Add1/1 -> Integrator/1  "dx2"
  1/M/1 -> Add1/5

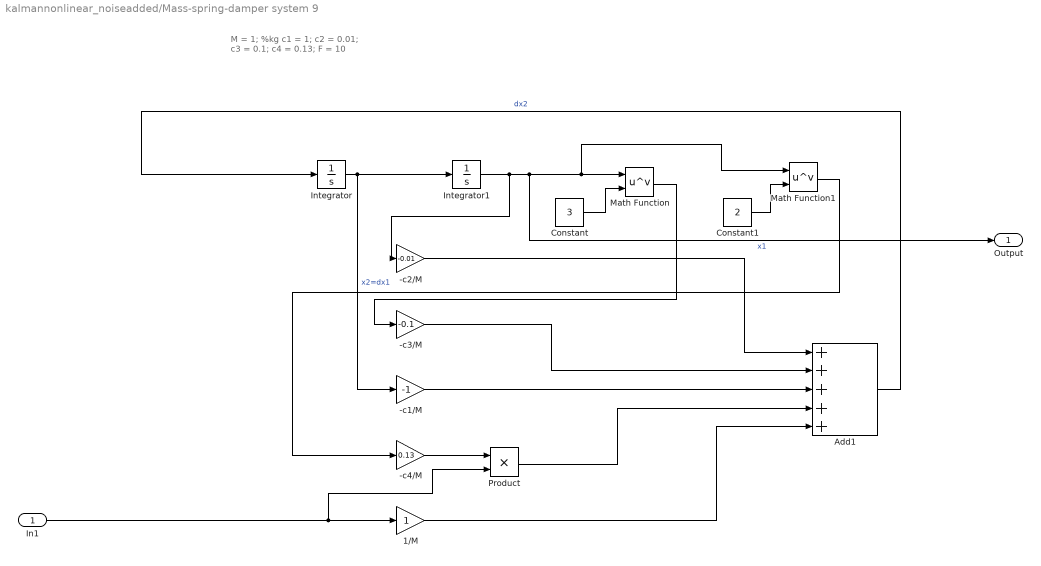
== system kalmannonlinear_noiseadded/Mass-spring-damper system 9 ==
  note: M  = 1; %kg
      | c1 = 1;
      | c2 = 0.01;
      | c3 = 0.1;
      | c4 = 0.13;
      | F  = 10
  In1 : Inport
  -c1/M : Gain  Gain=-1
  -c2/M : Gain  Gain=-0.01
  -c3/M : Gain  Gain=-0.1
  -c4/M : Gain  Gain=0.13
  1/M : Gain
  Add1 : Sum  Inputs=+++++
  Constant : Constant  Value=3
  Constant1 : Constant  Value=2
  Integrator : Integrator  InitialCondition=5
  Integrator1 : Integrator
  Math Function : Math  Operator=pow  SignedPower=off  SaturateOnIntegerOverflow=on
  Math Function1 : Math  Operator=pow  SignedPower=off  SaturateOnIntegerOverflow=on
  Product : Product
  Output : Outport
  wires:
  Integrator1/1 -> -c2/M/1, Output/1, Math Function1/1, Math Function/1  "x1"
  Math Function/1 -> -c3/M/1
  Constant/1 -> Math Function/2
  -c3/M/1 -> Add1/2
  Product/1 -> Add1/4
  -c1/M/1 -> Add1/3
  -c4/M/1 -> Product/1
  Math Function1/1 -> -c4/M/1
  Constant1/1 -> Math Function1/2
  -c2/M/1 -> Add1/1
  In1/1 -> Product/2, 1/M/1
  Integrator/1 -> -c1/M/1, Integrator1/1  "x2=dx1"
  Add1/1 -> Integrator/1  "dx2"
  1/M/1 -> Add1/5
